simulink model "Practical_Transformer"  (R2020a)
settings: Solver=ode45  StartTime=0.0  StopTime=0.2  RelTol=1e-3  EnableMultiTasking=on
values from neighbouring files (symbols this model uses):
  a = str2double(get(handles.edit75,'string'))    [PT_GUI.m]
  Eg = str2double(get(handles.edit67,'string'))    [PT_GUI.m]
  Ll = Xl/(2*pi*50)    [PT_GUI.m]
  Lm = Xm/(2*pi*50)    [PT_GUI.m]
  R = str2double(get(handles.edit68,'string'))    [PT_GUI.m]
  Rl = (Esc*Esc)/Psc    [PT_GUI.m]
  Rm = (Eoc*Eoc)/Poc    [PT_GUI.m]
libraries: powerlib x8, powerlib_meascontrol x5
settings Model: RequirementInfo="{}  %GIDa_bc8a8f9e_c6cb_4e4d_8f39_3b7530fd557f"  Creator=Karim Abouaish  LastModifiedBy=Emil
settings DataIOCC: ExternalInput=[t u]  LimitDataPoints=on  SaveFormat=Array  ReturnWorkspaceOutputs=off
settings OptimizationCC: LifeSpan=inf
settings DebuggingCC: UnderspecifiedInitializationDetection=Classic  MergeDetectMultiDrivingBlocksExec=none  SolverPrmCheckMsg=warning  StateNameClashWarn=warning  SFUnexpectedBacktrackingDiag=warning  SFNoUnconditionalDefaultTransitionDiag=warning  SFExecutionAtInitializationDiag=none  ArithmeticOperatorsInVariantConditions=warning
settings HardwareCC: ProdBitPerPointer=32  ProdBitPerSizeT=32  ProdBitPerPtrDiffT=32  ProdLargestAtomicFloat=None  ProdIntDivRoundTo=Undefined  ProdEndianess=Unspecified  ProdWordSize=32  ProdHWDeviceType=32-bit Generic
settings ModelReferenceCC: PropagateSignalLabelsOutOfModel=off
settings SFSimCC: SimUseLocalCustomCode=off  CustomCodeUndefinedFunction=UseInterfaceOnly
settings RTWCC: RTWUseLocalCustomCode=off
settings CodeAppCC: StateflowObjectComments=on
settings GRTTargetCC: TargetLangStandard=C89/C90 (ANSI)
settings ConfigComp: CovMetricSettings=dw  CovHtmlReporting=on  CovSaveCumulativeToWorkspaceVar=on  CovSaveSingleToWorkspaceVar=on  CovExternalEMLEnable=off
settings SimscapeCC: SimscapeNormalizeSystem=off

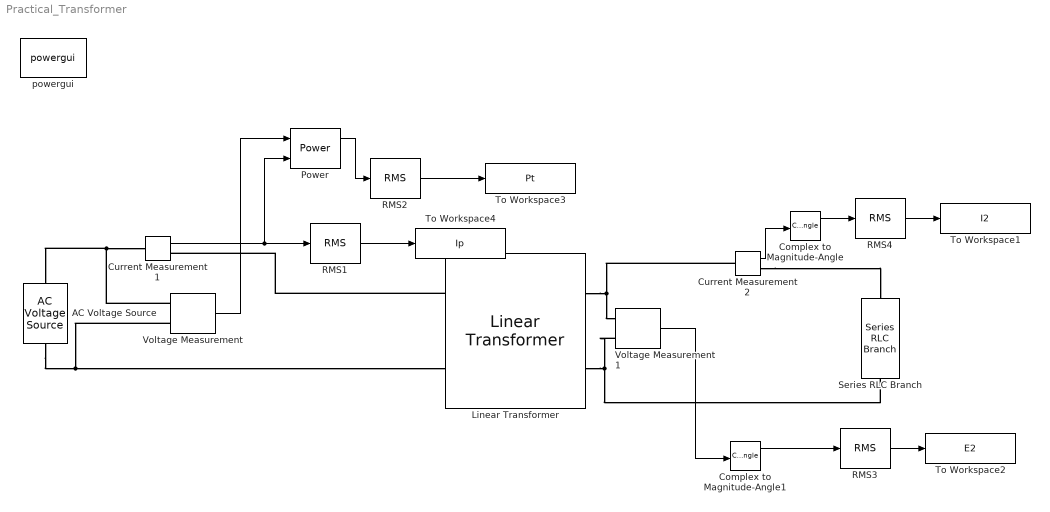
== system Practical_Transformer ==
  AC Voltage Source : powerlib/Electrical Sources/AC Voltage Source  Amplitude=Eg*sqrt(2)  Phase=0  Frequency=50  SampleTime=0  Measurements=None  BusType=swing  Pref=10e3  Qref=0  Qmin=-inf  Qmax=+inf
  Complex to Magnitude-Angle : ComplexToMagnitudeAngle
  Complex to Magnitude-Angle1 : ComplexToMagnitudeAngle
  Current Measurement1 : powerlib/Measurements/Current Measurement  PhasorSimulation=off  OutputType=Complex  PSBequivalent=0
  Current Measurement2 : powerlib/Measurements/Current Measurement  PhasorSimulation=off  OutputType=Complex  PSBequivalent=0
  Linear Transformer : powerlib/Elements/Linear Transformer  UNITS=SI  NominalPower=[ 250e6 50 ]  winding1=[a Rl Ll]  winding2=[1 0 0]  ThreeWindings=off  winding3=[3.15e+05 0.7938 0.084225]  RmLm=[Rm Lm]  Measurements=None  DataType=on
  Power : powerlib_meascontrol/Measurements/Power  Freq=50  Vinit=[1, 0]  Iinit=[1, 0]  Ts=0.001
  RMS{1..4} (4 alike) : powerlib_meascontrol/Measurements/RMS  TrueRMS=on  Freq=50  RMSInit=0  Ts=0.001
  Series RLC Branch : powerlib/Elements/Series RLC Branch  LConnTagsString=__new0  RConnTagsString=__new0  BranchType=RLC  Resistance=R  Inductance=0  SetiL0=off  InitialCurrent=0  Capacitance=0  Setx0=off  InitialVoltage=0  Measurements=None
  To Workspace1 : ToWorkspace  VariableName=I2  SampleTime=-1
  To Workspace2 : ToWorkspace  VariableName=E2  SampleTime=-1
  To Workspace3 : ToWorkspace  VariableName=Pt  SampleTime=-1
  To Workspace4 : ToWorkspace  VariableName=Ip  SampleTime=-1
  Voltage Measurement : powerlib/Measurements/Voltage Measurement  PhasorSimulation=off  OutputType=Complex  PSBequivalent=0
  Voltage Measurement1 : powerlib/Measurements/Voltage Measurement  PhasorSimulation=off  OutputType=Complex  PSBequivalent=0
  powergui : powerlib/powergui  Priority=1  SimulationMode=Continuous  SampleTime=50e-6  frequency=60  Iterations=50  frequencyindice=50  Pbase=100e6  ErrMax=1e-4  UnitsV=kV  UnitsW=MW  buscounter=0  FunctionMessages=off  echomessages=off  EnableUseOfTLC=off  CurrentSourceSwitches=off  DisableSnubberDevices=off  DisableRonSwitches=off  DisableVfSwitches=off  DisplayEquations=off  AutomaticDiscreteSolvers=off  SolverType=Tustin  Interpol=off  ExternalGateDelay=off  methode=off  Ts=0  x0status=blocks  SPID=off  SwTol=0  HookPort=off  NonlinearTolerance=1e-4  nMaxIteration=100  ContinueOnMaxIteration=off  RestoreLinks=warning  ResistiveCurrentMeasurement=off  Frange=[0:2:500]  Ylog=off  Xlog=on  ShowGrid=off  save=off  variable=ZData  structure=0  ZoomFFT=off  StartTime=0.0  cycles=1  DisplayStyle=1  fundamental=60  FreqAxis=off  MaxFrequency=1000  frequencyindicesteady=1  RmsSteady=1  display=off
  wires:
  Current Measurement1/1 -> Power/2, RMS1/1
  RMS1/1 -> To Workspace4/1
  Voltage Measurement/1 -> Power/1
  Power/1 -> RMS2/1
  RMS2/1 -> To Workspace3/1
  RMS4/1 -> To Workspace1/1
  RMS3/1 -> To Workspace2/1
  Current Measurement2/1 -> Complex to Magnitude-Angle/1
  Complex to Magnitude-Angle/1 -> RMS4/1
  Voltage Measurement1/1 -> Complex to Magnitude-Angle1/1
  Complex to Magnitude-Angle1/1 -> RMS3/1
  connections:
  Voltage Measurement/LConn1 -- Current Measurement1/LConn1 -- AC Voltage Source/RConn1
  AC Voltage Source/LConn1 -- Linear Transformer/LConn2 -- Voltage Measurement/LConn2
  Linear Transformer/LConn1 -- Current Measurement1/RConn1
  Linear Transformer/RConn1 -- Current Measurement2/LConn1 -- Voltage Measurement1/LConn1
  Linear Transformer/RConn2 -- Voltage Measurement1/LConn2 -- Series RLC Branch/RConn1
  Current Measurement2/RConn1 -- Series RLC Branch/LConn1
